simulink model "MS_alpha_beta"  (R2014a)
settings: Solver=ode3  StartTime=0.0  StopTime=100  FixedStep=0.0001  RelTol=1e-3
values from neighbouring files (symbols this model uses):
  ClarkConcordia = sqrt(3/2)*[1 -1/2 -1/2; 0 sqrt(3)/2 -sqrt(3)/2; 1/sqrt(2) 1/sqrt(2) 1/sqrt(2)]    [MS_alpha_beta_.m]
  f = 0    [MS_alpha_beta_.m]
  fe = 2.3036    [MS_alpha_beta_.m]
  J = 0.00529    [MS_alpha_beta_.m]
  L0 = (Ld+Lq)/2    (= 0.86431)    [MS_alpha_beta_.m]
  L2 = (Ld-Lq)/2    (= 0)    [MS_alpha_beta_.m]
  Ld = 0.86431    [MS_alpha_beta_.m]
  Lq = 0.86431    [MS_alpha_beta_.m]
  Rs = 0.032988    [MS_alpha_beta_.m]
  Vs = 1    [MS_alpha_beta_.m]
settings Model: Creator=User  LastModifiedBy=User

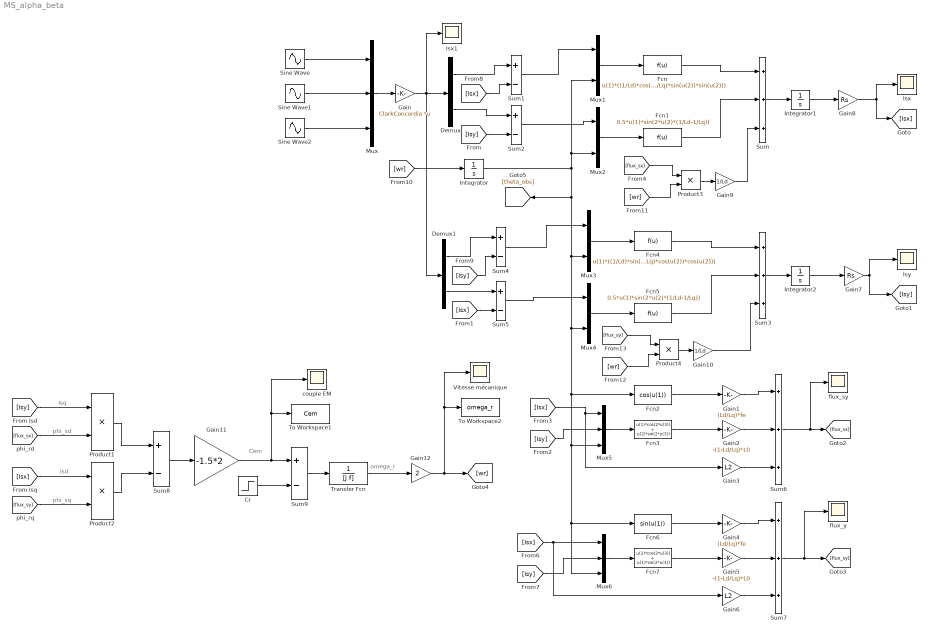
== system MS_alpha_beta ==
  note: Isq
  note: phi_sd
  note: phi_sq
  note: Isd
  note: omega_r
  note: Cem
  Cr : Step  Time=300  After=0.1  SampleTime=0
  Demux : Demux  Outputs=2
  Demux1 : Demux  Outputs=2
  Fcn : Fcn  Expr=u(1)*((1/Ld)*cos(u(2))*cos(u(2)) + (1/Lq)*sin(u(2))*sin(u(2)))
  Fcn1 : Fcn  Expr=0.5*u(1)*sin(2*u(2)*(1/Ld-1/Lq))
  Fcn2 : Fcn  Expr=cos(u(1))
  Fcn3 : Fcn  Expr=u(1)*cos(2*u(3)) + u(2)*sin(2*u(3))
  Fcn4 : Fcn  Expr=u(1)*((1/Ld)*sin(u(2))*sin(u(2)) + (1/Lq)*cos(u(2))*cos(u(2)))
  Fcn5 : Fcn  Expr=0.5*u(1)*sin(2*u(2)*(1/Ld-1/Lq))
  Fcn6 : Fcn  Expr=sin(u(1))
  Fcn7 : Fcn  Expr=u(2)*cos(2*u(3)) + u(1)*sin(2*u(3))
  Gain : Gain  Gain=ClarkConcordia  Multiplication=Matrix(K*u)
  Gain1 : Gain  Gain=(Ld/Lq)*fe
  Gain10 : Gain  Gain=1/Ld
  Gain11 : Gain  Gain=-1.5*2
  Gain12 : Gain  Gain=2
  Gain2 : Gain  Gain=-(1-Ld/Lq)*L0
  Gain3 : Gain  Gain=L2
  Gain4 : Gain  Gain=(Ld/Lq)*fe
  Gain5 : Gain  Gain=-(1-Ld/Lq)*L0
  Gain6 : Gain  Gain=L2
  Gain7 : Gain  Gain=Rs
  Gain8 : Gain  Gain=Rs
  Gain9 : Gain  Gain=1/Ld
  Integrator : Integrator
  Integrator1 : Integrator
  Integrator2 : Integrator
  Isx : Scope
  Isx1 : Scope
      settings: SaveName=ScopeData6
  Isy : Scope
      settings: YMin=-500  YMax=500
  Mux : Mux  Inputs=3
  Mux{1..4} (4 alike) : Mux  Inputs=2
  Mux5 : Mux  Inputs=3
  Mux6 : Mux  Inputs=3
  Product{1..4} (4 alike) : Product
  Sine Wave : Sin  Amplitude=Vs  Frequency=0.1  SampleTime=0
  Sine Wave1 : Sin  Amplitude=Vs  Frequency=0.1  Phase=-2*pi/3  SampleTime=0
  Sine Wave2 : Sin  Amplitude=Vs  Frequency=0.1  Phase=-4*pi/3  SampleTime=0
  Sum{,3,6..7} (4 alike) : Sum  Inputs=+++
  Sum{1..2,4..5,8..9} (6 alike) : Sum  Inputs=+-
  To Workspace1 : ToWorkspace  VariableName=Cem  SaveFormat=Timeseries  SampleTime=-1
  To Workspace2 : ToWorkspace  VariableName=omega_r  SaveFormat=Timeseries  SampleTime=-1
  Transfer Fcn : TransferFcn  Denominator=[J f]
  Vitesse mécanique : Scope
      settings: YMin=-25  YMax=22.5  SaveName=ScopeData2
  couple EM : Scope
      settings: SaveName=ScopeData3
  flux_sy : Scope
      settings: SaveName=ScopeData4
  flux_y : Scope
      settings: SaveName=ScopeData5
  wires:
  Sine Wave/1 -> Mux/1
  Sine Wave1/1 -> Mux/2
  Sine Wave2/1 -> Mux/3
  Mux/1 -> Gain/1
  Gain/1 -> Isx1/1, Demux/1, Demux1/1
  [wr] -> Integrator/1
  Mux1/1 -> Fcn/1
  Mux2/1 -> Fcn1/1
  Fcn/1 -> Sum/1
  Fcn1/1 -> Sum/2
  Sum/1 -> Integrator1/1
  Demux/1 -> Sum1/1
  Demux/2 -> Sum2/1
  Sum1/1 -> Mux1/1
  Sum2/1 -> Mux2/1
  Fcn2/1 -> Gain1/1
  Fcn3/1 -> Gain2/1
  Mux3/1 -> Fcn4/1
  Mux4/1 -> Fcn5/1
  Fcn4/1 -> Sum3/1
  Fcn5/1 -> Sum3/2
  Sum3/1 -> Integrator2/1
  Sum4/1 -> Mux3/1
  Sum5/1 -> Mux4/1
  Demux1/1 -> Sum4/1
  Demux1/2 -> Sum5/1
  Mux5/1 -> Fcn3/1
  [Isx] -> Sum5/2
  [Isx] -> Gain3/1, Mux5/1
  [Isy] -> Mux5/2
  Gain1/1 -> Sum6/1
  Gain2/1 -> Sum6/2
  Gain3/1 -> Sum6/3
  Fcn6/1 -> Gain4/1
  Fcn7/1 -> Gain5/1
  Integrator/1 -> Mux2/2, Mux1/2, [theta_obs], Fcn6/1, Mux6/3, Mux5/3, Fcn2/1, Mux4/2, Mux3/2
  Mux6/1 -> Fcn7/1
  [Isx] -> Mux6/1, Gain6/1
  [Isy] -> Mux6/2
  Gain4/1 -> Sum7/1
  Gain5/1 -> Sum7/2
  Gain6/1 -> Sum7/3
  Integrator2/1 -> Gain7/1
  Gain7/1 -> [Isy], Isy/1
  Integrator1/1 -> Gain8/1
  Gain8/1 -> [Isx], Isx/1
  [Isx] -> Sum1/2
  [Isy] -> Sum4/2
  Sum6/1 -> flux_sy/1, [flux_sx]
  Sum7/1 -> flux_y/1, [flux_sy]
  Gain11/1 -> To Workspace1/1, couple EM/1, Sum9/1
  Transfer Fcn/1 -> Gain12/1
  [Isx] -> Product2/1
  [flux_sy] -> Product2/2
  [flux_sx] -> Product1/2
  Sum9/1 -> Transfer Fcn/1
  Sum8/1 -> Gain11/1
  Cr/1 -> Sum9/2
  Product2/1 -> Sum8/2
  [Isy] -> Product1/1
  Gain12/1 -> To Workspace2/1, Vitesse mécanique/1, [wr]
  Product1/1 -> Sum8/1
  [Isy] -> Sum2/2
  [wr] -> Product3/2
  [flux_sx] -> Product3/1
  Product3/1 -> Gain9/1
  Gain9/1 -> Sum/3
  [wr] -> Product4/2
  [flux_sy] -> Product4/1
  Product4/1 -> Gain10/1
  Gain10/1 -> Sum3/3
